simulink model "Walsh04Class_homeAllSignal"  (R2021a)
settings: Solver=VariableStepAuto  StartTime=0.0  StopTime=96  RelTol=1e-3
settings Model: Creator=alexandr.lanin  LastModifiedBy=Alex
settings SolverCC: AlgebraicLoopSolver=TrustRegion
settings DataIOCC: ReturnWorkspaceOutputs=off
settings DebuggingCC: SFMachineParentedDataDiag=warning  ArithmeticOperatorsInVariantConditions=warning
settings SFSimCC: SimUseLocalCustomCode=off  CustomCodeUndefinedFunction=UseInterfaceOnly
settings RTWCC: RTWUseLocalCustomCode=off
settings CodeAppCC: StateflowObjectComments=on

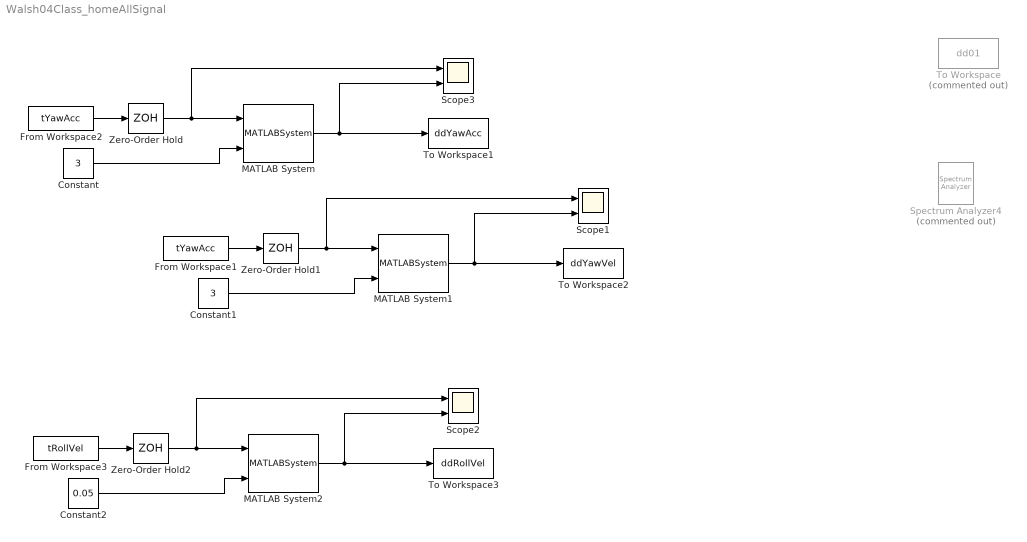
== system Walsh04Class_homeAllSignal ==
  Constant : Constant  Value=3
  Constant1 : Constant  Value=3
  Constant2 : Constant  Value=0.05
  From Workspace1 : FromWorkspace  VariableName=tYawAcc
  From Workspace2 : FromWorkspace  VariableName=tYawAcc
  From Workspace3 : FromWorkspace  VariableName=tRollVel
  MATLAB System : MATLABSystem  System=WolchSim  SimulateUsing=Code generation
      mask Type: WolchSim
      mask Display:
      | disp('WolchSim');
      | port_label('input',1,'u');
      | port_label('input',2,'norm');
      | port_label('output',1,'y');
  MATLAB System1 : MATLABSystem  System=WolchSim  SimulateUsing=Code generation
      mask Type: WolchSim
      mask Display:
      | disp('WolchSim');
      | port_label('input',1,'u');
      | port_label('input',2,'norm');
      | port_label('output',1,'y');
  MATLAB System2 : MATLABSystem  System=WolchSim  SimulateUsing=Code generation
      mask Type: WolchSim
      mask Display:
      | disp('WolchSim');
      | port_label('input',1,'u');
      | port_label('input',2,'norm');
      | port_label('output',1,'y');
  Scope1 : Scope  NumInputPorts=2
  Scope2 : Scope  NumInputPorts=2
  Scope3 : Scope  NumInputPorts=2
  Spectrum Analyzer4 : SpectrumAnalyzer  Commented=on
  To Workspace : ToWorkspace  Commented=on  VariableName=dd01  SaveFormat=Timeseries  SampleTime=-1
  To Workspace1 : ToWorkspace  VariableName=ddYawAcc  SaveFormat=Timeseries  SampleTime=-1
  To Workspace2 : ToWorkspace  VariableName=ddYawVel  SaveFormat=Timeseries  SampleTime=-1
  To Workspace3 : ToWorkspace  VariableName=ddRollVel  SaveFormat=Timeseries  SampleTime=-1
  Zero-Order Hold : ZeroOrderHold  SampleTime=0.01
  Zero-Order Hold1 : ZeroOrderHold  SampleTime=0.01
  Zero-Order Hold2 : ZeroOrderHold  SampleTime=0.01
  wires:
  From Workspace2/1 -> Zero-Order Hold/1
  Zero-Order Hold/1 -> Scope3/1, MATLAB System/1
  Constant/1 -> MATLAB System/2
  MATLAB System/1 -> To Workspace1/1, Scope3/2
  Constant1/1 -> MATLAB System1/2
  MATLAB System1/1 -> To Workspace2/1, Scope1/2
  Zero-Order Hold1/1 -> Scope1/1, MATLAB System1/1
  From Workspace1/1 -> Zero-Order Hold1/1
  Constant2/1 -> MATLAB System2/2
  MATLAB System2/1 -> To Workspace3/1, Scope2/2
  Zero-Order Hold2/1 -> Scope2/1, MATLAB System2/1
  From Workspace3/1 -> Zero-Order Hold2/1
